simulink model "ACFT"  (R2024b)
settings: Solver=VariableStepAuto  StartTime=0.0  StopTime=10.0  RelTol=1e-3
values from neighbouring files (symbols this model uses):
  alfa_deg = -1.8    [initACFT_high.m]    (also in init_Cessna.m = 1)
  b = params.b    [Aerodynamics_Coefficient.m]    (also in AeroforcesandMoments.m; initACFT_high.m = 21; initACFT_low.m = 21; init_Cessna.m = 10.9728)
  c = params.c    [Aerodynamics_Coefficient.m]    (also in AeroforcesandMoments.m; initACFT_high.m = 2.5; initACFT_low.m = 2.5; init_Cessna.m = 1.49352)
  CD0 = params.CD0    [Aerodynamics_Coefficient.m]    (also in initACFT_high.m = 0.0281; initACFT_low.m = 0.023; init_Cessna.m = 0.027)
  CD_alpha = params.CD_alpha    [Aerodynamics_Coefficient.m]    (also in initACFT_high.m = 0.5157; initACFT_low.m = 0.1318; init_Cessna.m = 0.26)
  CD_elev = params.CD_elev    [Aerodynamics_Coefficient.m]    (also in initACFT_high.m = 0.0178; initACFT_low.m = 0.0178; init_Cessna.m = 0)
  CI_beta = params.CI_beta    [Aerodynamics_Coefficient.m]
  CI_p = params.CI_p    [Aerodynamics_Coefficient.m]
  CI_r = params.CI_r    [Aerodynamics_Coefficient.m]
  CI_rud = params.CI_rud    [Aerodynamics_Coefficient.m]
  CL0 = params.CL0    [Aerodynamics_Coefficient.m]    (also in initACFT_high.m = 0.209; initACFT_low.m = 0.19; init_Cessna.m = 0.307)
  CL_alpha = params.CL_alpha    [Aerodynamics_Coefficient.m]    (also in initACFT_high.m = 8.7491; initACFT_low.m = 6.1879; init_Cessna.m = 4.41)
  CL_elev = params.CL_elev    [Aerodynamics_Coefficient.m]    (also in initACFT_high.m = 0.538; initACFT_low.m = 0.4727; init_Cessna.m = 0.43)
  CL_q = params.CL_q    [Aerodynamics_Coefficient.m]    (also in initACFT_high.m = 4.14; initACFT_low.m = 4.66; init_Cessna.m = 3.9)
  Cm0 = params.Cm0    [Aerodynamics_Coefficient.m]    (also in initACFT_high.m = 0; initACFT_low.m = 0.0133; init_Cessna.m = 0.04)
  Cm_alpha = params.Cm_alpha    [Aerodynamics_Coefficient.m]    (also in initACFT_high.m = -2.4351; initACFT_low.m = -2.0168; init_Cessna.m = -0.613)
  Cm_AlphaDot = params.Cm_AlphaDot    [Aerodynamics_Coefficient.m]    (also in initACFT_high.m = -4.53; initACFT_low.m = -6.76; init_Cessna.m = -7.27)
  Cm_elev = params.Cm_elev    [Aerodynamics_Coefficient.m]    (also in initACFT_high.m = -1.9079; initACFT_low.m = -1.6788; init_Cessna.m = -1.122)
  Cm_q = params.Cm_q    [Aerodynamics_Coefficient.m]    (also in initACFT_high.m = -37.6; initACFT_low.m = -36.3; init_Cessna.m = -12.4)
  Cn_ail = -8.5944e-04    (= -0.00085944)    [initACFT_high.m]    (also in initACFT_low.m = -0.00063025; init_Cessna.m = -0.0216)
  Cn_beta = 0.1478    [initACFT_high.m]    (also in initACFT_low.m = 0.1209; init_Cessna.m = 0.0587)
  Cn_p = -0.114    [initACFT_high.m]    (also in initACFT_low.m; init_Cessna.m = -0.0278)
  Cn_r = -0.15    [initACFT_high.m]    (also in initACFT_low.m = -0.3; init_Cessna.m = -0.0937)
  Cn_rud = -0.1100    (= -0.11)    [initACFT_high.m]    (also in initACFT_low.m = -0.102; init_Cessna.m = -0.0645)
  CY_ail = 0    [initACFT_high.m]    (also in initACFT_low.m; init_Cessna.m)
  CY_beta = params.CY_beta    [Aerodynamics_Coefficient.m]    (also in initACFT_high.m = -1.2777; initACFT_low.m = -1.1803; init_Cessna.m = -0.404)
  CY_p = params.CY_p    [Aerodynamics_Coefficient.m]    (also in initACFT_high.m = 0.3; initACFT_low.m = 0.3; init_Cessna.m = -0.075)
  CY_r = params.CY_r    [Aerodynamics_Coefficient.m]    (also in initACFT_high.m = 0.91; initACFT_low.m = 0.91; init_Cessna.m = 0.214)
  CY_rud = params.CY_rud    [Aerodynamics_Coefficient.m]    (also in initACFT_high.m = 0.4343; initACFT_low.m = 0.4016; init_Cessna.m = 0.187)
  Inertia = [Ixx 0 -Ixz; 0 Iyy 0; -Ixz 0 Izz]    [initACFT_high.m]    (also in initACFT_low.m; init_Cessna.m)
  nrho = 0.75    [initACFT_high.m]    (also in initACFT_low.m; init_Cessna.m)
  nv = 0    [initACFT_high.m]    (also in initACFT_low.m; init_Cessna.m = -1)
  rho_reference_kgpm3 = 1.225    [initACFT_high.m]    (also in init_Cessna.m)
  S = 45    [initACFT_high.m]    (also in initACFT_low.m; init_Cessna.m = 16.2)
  V_reference_mps = 200    [initACFT_high.m]    (also in init_Cessna.m = 51.4)
  xf_m = -3.8    [initACFT_high.m]    (also in initACFT_low.m; init_Cessna.m = 1)
  z_cg = -0.4    [initACFT_high.m]    (also in initACFT_low.m; init_Cessna.m = 0.2)
  zf_m = -0.6    [initACFT_high.m]    (also in initACFT_low.m; init_Cessna.m = 0)
undefined symbols (not defined in the file or in its folder): CI_ail, CL_AlphaDot_, TMax, Y_cg, Z_cg

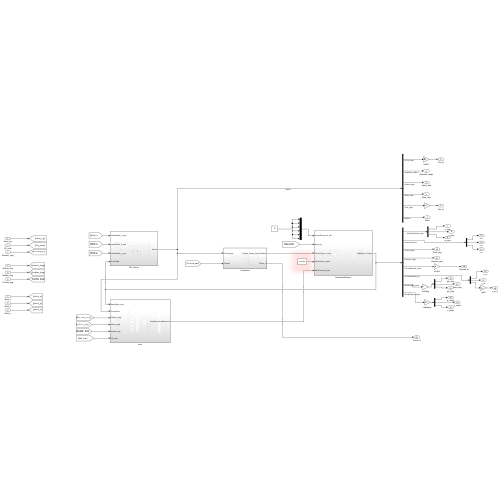
[thumbnail: Simulink's stored preview of the top-level diagram]
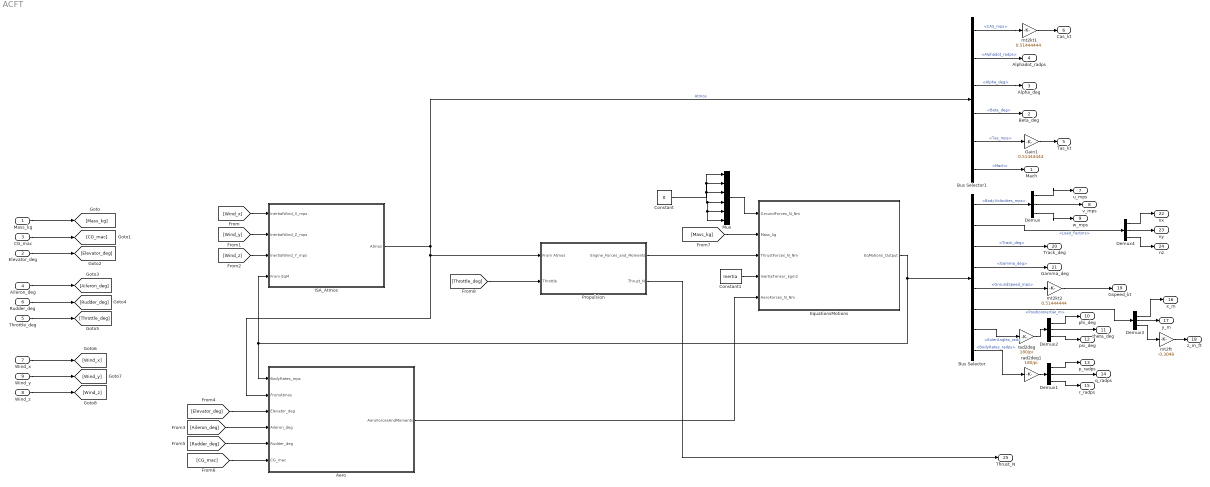
== system ACFT ==
  Mass_kg : Inport
  Elevator_deg : Inport  Port=2
  CG_mac : Inport  Port=3
  Aileron_deg : Inport  Port=4
  Throttle_deg : Inport  Port=5
  Rudder_deg : Inport  Port=6
  Wind_x : Inport  Port=7
  Wind_z : Inport  Port=8
  Wind_y : Inport  Port=9
  Aero : Subsystem
  Bus Selector : BusSelector  OutputSignals=BodyVolocities_mps,Load_Factors,Track_deg,Gamma_deg,GroundSpeed_mps,PositionInertial_m,EulerAngles_rad,BodyRates_radps
  Bus Selector1 : BusSelector  OutputSignals=CAS_mps,Alphadot_radps,Alpha_deg,Beta_deg,Tas_mps,Mach
  Constant : Constant  Value=0
  Constant1 : Constant  Value=Inertia
  Demux{,1..4} (5 alike) : Demux  Outputs=3
  EquationsMotions : Subsystem
  Gain1 : Gain  Gain=0.51444444
  ISA_Atmos : Subsystem
  Mux : Mux  Inputs=6
  Propulsion : Subsystem
  mt2ft : Gain  Gain=-0.3048
  mt2kt1 : Gain  Gain=0.51444444
  mt2kt2 : Gain  Gain=0.51444444
  rad2deg : Gain  Gain=180/pi
  rad2deg1 : Gain  Gain=180/pi
  Mach : Outport
  Beta_deg : Outport  Port=2
  Alpha_deg : Outport  Port=3
  Alphadot_radps : Outport  Port=4
  Tas_kt : Outport  Port=5
  Cas_kt : Outport  Port=6
  u_mps : Outport  Port=7
  v_mps : Outport  Port=8
  w_mps : Outport  Port=9
  phi_deg : Outport  Port=10
  theta_deg : Outport  Port=11
  psi_deg : Outport  Port=12
  p_radps : Outport  Port=13
  q_radps : Outport  Port=14
  r_radps : Outport  Port=15
  x_m : Outport  Port=16
  y_m : Outport  Port=17
  z_m_ft : Outport  Port=18
  Gspeed_kt : Outport  Port=19
  Track_deg : Outport  Port=20
  Gamma_deg : Outport  Port=21
  nx : Outport  Port=22
  ny : Outport  Port=23
  nz : Outport  Port=24
  Thrust_N : Outport  Port=25
  wires:
  EquationsMotions/1(EqMotions_Output) -> Aero/1(BodyRates_mps), ISA_Atmos/4(From EqM), Bus Selector/1
  ISA_Atmos/1(Atmos) -> Aero/2(FromAtmos), Propulsion/1(From Atmos), Bus Selector1/1  "Atmos"
  Aero/1(AeroForcesAndMoments) -> EquationsMotions/5(AeroForces_N_Nm)
  Propulsion/2(Thrust_N) -> Thrust_N/1
  Constant/1 -> Mux/1, Mux/6, Mux/5, Mux/4, Mux/3, Mux/2
  Mux/1 -> EquationsMotions/1(GroundForces_N_Nm)
  Constant1/1 -> EquationsMotions/4(InertiaTensor_kgm2)
  CG_mac/1 -> [CG_mac]
  Aileron_deg/1 -> [Aileron_deg]
  Rudder_deg/1 -> [Rudder_deg]
  Wind_x/1 -> [Wind_x]
  Wind_y/1 -> [Wind_y]
  Wind_z/1 -> [Wind_z]
  Throttle_deg/1 -> [Throttle_deg]
  Elevator_deg/1 -> [Elevator_deg]
  Mass_kg/1 -> [Mass_kg]
  [Wind_x] -> ISA_Atmos/1(InertialWind_X_mps)
  [Wind_y] -> ISA_Atmos/2(InertialWind_Z_mps)
  [Wind_z] -> ISA_Atmos/3(InertialWind_Y_mps)
  [Aileron_deg] -> Aero/4(Aileron_deg)
  [Elevator_deg] -> Aero/3(Elevator_deg)
  [Rudder_deg] -> Aero/5(Rudder_deg)
  [CG_mac] -> Aero/6(CG_mac)
  [Mass_kg] -> EquationsMotions/2(Mass_kg)
  [Throttle_deg] -> Propulsion/2(Throttle)
  Bus Selector1/1 -> mt2kt1/1  "<CAS_mps>"
  Bus Selector1/2 -> Alphadot_radps/1  "<Alphadot_radps>"
  Bus Selector1/3 -> Alpha_deg/1  "<Alpha_deg>"
  Bus Selector1/4 -> Beta_deg/1  "<Beta_deg>"
  Bus Selector1/5 -> Gain1/1  "<Tas_mps>"
  Bus Selector1/6 -> Mach/1  "<Mach>"
  Gain1/1 -> Tas_kt/1
  mt2kt1/1 -> Cas_kt/1
  Bus Selector/1 -> Demux/1  "<BodyVolocities_mps>"
  Bus Selector/3 -> Track_deg/1  "<Track_deg>"
  Bus Selector/4 -> Gamma_deg/1  "<Gamma_deg>"
  Bus Selector/6 -> Demux3/1  "<PositionInertial_m>"
  Bus Selector/7 -> rad2deg/1  "<EulerAngles_rad>"
  Bus Selector/8 -> rad2deg1/1  "<BodyRates_radps>"
  rad2deg/1 -> Demux2/1
  rad2deg1/1 -> Demux1/1
  Demux/1 -> u_mps/1
  Demux/3 -> w_mps/1
  Demux/2 -> v_mps/1
  Demux2/2 -> theta_deg/1
  Demux2/1 -> phi_deg/1
  Demux2/3 -> psi_deg/1
  Demux1/1 -> p_radps/1
  Demux1/3 -> r_radps/1
  Demux1/2 -> q_radps/1
  Demux3/2 -> y_m/1
  Demux3/1 -> x_m/1
  Demux3/3 -> mt2ft/1
  mt2ft/1 -> z_m_ft/1
  Bus Selector/5 -> mt2kt2/1  "<GroundSpeed_mps>"
  mt2kt2/1 -> Gspeed_kt/1
  Bus Selector/2 -> Demux4/1  "<Load_Factors>"
  Demux4/1 -> nx/1
  Demux4/3 -> nz/1
  Demux4/2 -> ny/1
  Propulsion/1(Engine_Forces_and_Moments) -> EquationsMotions/3(ThrustForces_N_Nm)

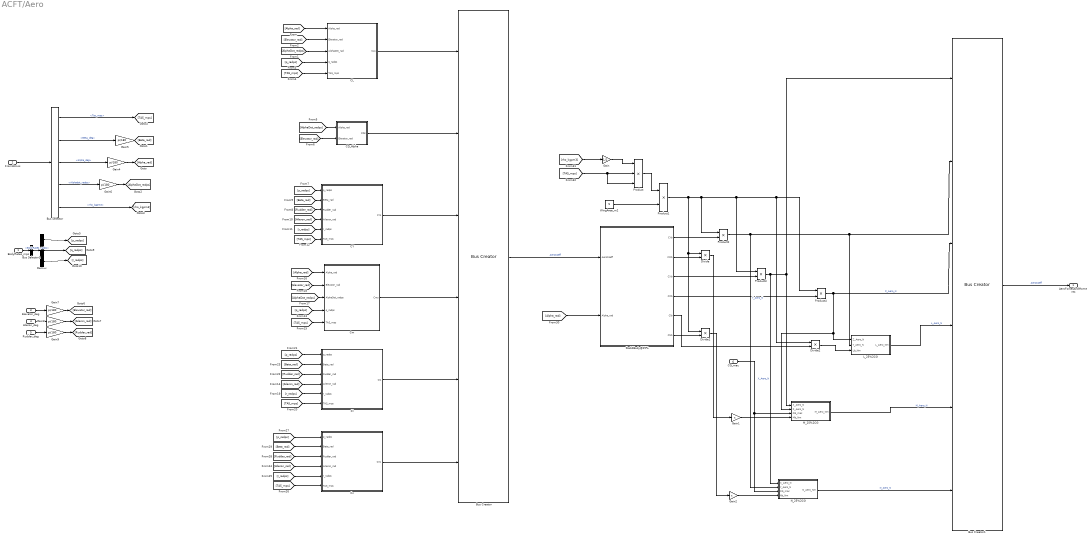
== system ACFT/Aero ==
  BodyRates_mps : Inport
  FromAtmos : Inport  Port=2
  Elevator_deg : Inport  Port=3
  Aileron_deg : Inport  Port=4
  Rudder_deg : Inport  Port=5
  CG_mac : Inport  Port=6
  Bus Creator : BusCreator  Inputs=6
  Bus Creator1 : BusCreator  Inputs=6
  Bus Selector : BusSelector  OutputSignals=Tas_mps,Beta_deg,Alpha_deg,Alphadot_radps,rho_kgpm3
  Bus Selector1 : BusSelector  OutputSignals=BodyRates_radps
  CD_Alpha : Subsystem
  CI : Subsystem
  CL : Subsystem
  CY : Subsystem
  Cm : Subsystem
  Cn : Subsystem
  Demux : Demux  Outputs=3
  Divide : Product
  Divide1 : Product
  Divide2 : Product
  Gain : Gain  Gain=1/2
  Gain1 : Gain  Gain=c
  Gain2 : Gain  Gain=c
  Gain{4..9} (6 alike) : Gain  Gain=pi/180
  L_25%2CG : Subsystem
  M_25%2CG : Subsystem
  N_25%2CG : Subsystem
  Product : Product  Inputs=3
  Product{1..4} (4 alike) : Product
  Stab2Body@25% : Subsystem
  WingArea_m2 : Constant  Value=S
  AeroForcesAndMoments : Outport
  wires:
  [p_radps] -> Cn/1(p_radps)
  [r_radps] -> CI/5(r_radps)
  Stab2Body@25%/2(CMb) -> Divide/2
  Stab2Body@25%/5(Clb) -> Divide2/2
  [rho_kgpm3] -> Gain/1
  Gain7/1 -> [Elevator_rad]
  Gain6/1 -> [AlphaDot_radps]
  CL/1(CLs) -> Bus Creator/1
  [TAS_mps] -> Cn/6(TAS_mps)
  [AlphaDot_radps] -> CL/3(AlphaDot_rad)
  N_25%2CG/1(N_Aero_Nm) -> Bus Creator1/6  "N_Aero_N"
  CI/1(CIs) -> Bus Creator/5
  M_25%2CG/1(M_Aero_Nm) -> Bus Creator1/5  "M_Aero_N"
  [p_radps] -> CY/1(p_radps)
  Stab2Body@25%/4(CZb) -> Product4/2
  [Alpha_rad] -> CL/1(Alpha_rad)
  [Aileron_rad] -> CI/4(Aileron_rad)
  Gain5/1 -> [Beta_rad]
  Cm/1(Cms) -> Bus Creator/4
  Gain2/1 -> N_25%2CG/4(Nb_Nm)
  [Beta_rad] -> CY/2(Beta_rad)
  Product2/1 -> L_25%2CG/2(Y_Aero_N), Bus Creator1/2, N_25%2CG/2(Y_Aero_N)  "Y_Aero_N"
  Elevator_deg/1 -> Gain7/1
  Gain/1 -> Product/1
  [Aileron_rad] -> Cn/4(Aileron_rad)
  CG_mac/1 -> M_25%2CG/3(CG_mac), N_25%2CG/3(CG_mac)
  [Rudder_rad] -> Cn/3(Rudder_rad)
  Demux/2 -> [q_radps]
  CD_Alpha/1(CDs) -> Bus Creator/2
  Demux/1 -> [p_radps]
  [TAS_mps] -> Cm/5(TAS_mps)
  [TAS_mps] -> Product/2, Product/3
  L_25%2CG/1(L_Aero_Nm) -> Bus Creator1/4  "L_Aero_N"
  Demux/3 -> [r_radps]
  CY/1(CYs) -> Bus Creator/3
  [AlphaDot_radps] -> Cm/3(AlphaDot_radps)
  [Rudder_rad] -> CI/3(Rudder_rad)
  [p_radps] -> CI/1(p_radps)
  [Rudder_rad] -> CY/3(Rudder_rad)
  Product1/1 -> Divide2/1, Product4/1, Product3/1, Product2/1, Divide/1, Divide1/1
  Gain1/1 -> M_25%2CG/4(Mb_Nm)
  Product4/1 -> Bus Creator1/3, L_25%2CG/1(Z_Aero_N), M_25%2CG/2(Z_Aero_N)  "Z_Aero_N"
  [Elevator_rad] -> Cm/2(Elevator_rad)
  Divide2/1 -> L_25%2CG/3(Lb_Nm)
  Gain9/1 -> [Rudder_rad]
  Aileron_deg/1 -> Gain8/1
  [Alpha_rad] -> Cm/1(Alpha_rad)
  Gain8/1 -> [Aileron_rad]
  [Beta_rad] -> Cn/2(Beta_rad)
  [Elevator_rad] -> CD_Alpha/2(Elevator_rad)
  Stab2Body@25%/1(CYb) -> Product2/2
  Rudder_deg/1 -> Gain9/1
  [Elevator_rad] -> CL/2(Elevator_rad)
  [Alpha_rad] -> Stab2Body@25%/2(Alpha_rad)
  Gain4/1 -> [Alpha_rad]
  Bus Creator/1 -> Stab2Body@25%/1(AeroCoeff)  "AeroCoeff"
  Stab2Body@25%/6(CNb) -> Divide1/2
  Cn/1(Cns) -> Bus Creator/6
  WingArea_m2/1 -> Product1/2
  [Aileron_rad] -> CY/4(Aileron_rad)
  [TAS_mps] -> CL/5(TAS_mps)
  Product/1 -> Product1/1
  Stab2Body@25%/3(CXb) -> Product3/2
  [AlphaDot_radps] -> CD_Alpha/1(Alpha_rad)
  Product3/1 -> Bus Creator1/1, M_25%2CG/1(X_Aero_N), N_25%2CG/1(X_Aero_N)  "X_Aero_N"
  [Beta_rad] -> CI/2(Beta_rad)
  [TAS_mps] -> CI/6(TAS_mps)
  [r_radps] -> CY/5(r_radps)
  Bus Creator1/1 -> AeroForcesAndMoments/1  "AeroCoeff"
  Divide1/1 -> Gain2/1
  [q_radps] -> Cm/4(q_radps)
  [TAS_mps] -> CY/6(TAS_mps)
  Divide/1 -> Gain1/1
  [r_radps] -> Cn/5(r_radps)
  [q_radps] -> CL/4(q_radps)
  FromAtmos/1 -> Bus Selector/1
  Bus Selector/2 -> Gain5/1  "<Beta_deg>"
  Bus Selector/3 -> Gain4/1  "<Alpha_deg>"
  Bus Selector/4 -> Gain6/1  "<Alphadot_radps>"
  Bus Selector/5 -> [rho_kgpm3]  "<rho_kgpm3>"
  Bus Selector/1 -> [TAS_mps]  "<Tas_mps>"
  BodyRates_mps/1 -> Bus Selector1/1
  Bus Selector1/1 -> Demux/1  "<BodyRates_radps>"

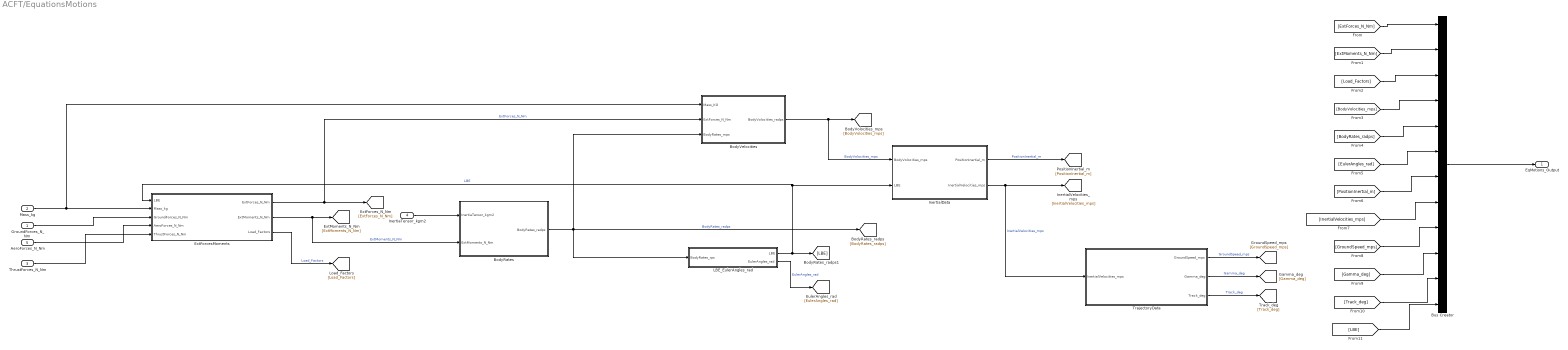
== system ACFT/EquationsMotions ==
  GroundForces_N_Nm : Inport
  Mass_kg : Inport  Port=2
  ThrustForces_N_Nm : Inport  Port=3
  InertiaTensor_kgm2 : Inport  Port=4
  AeroForces_N_Nm : Inport  Port=5
  BodyRates : Subsystem
  BodyVelocities : Subsystem
  Bus Creator : BusCreator  Inputs=12
  ExtForcesMoments : Subsystem
  InertialData : Subsystem
  LBE_EulerAngles_rad : Subsystem
  TrajectoryData : Subsystem
  EqMotions_Output : Outport
  wires:
  [Track_deg] -> Bus Creator/11
  [InertialVelocities_mps] -> Bus Creator/8
  [GroundSpeed_mps] -> Bus Creator/9
  [EulerAngles_rad] -> Bus Creator/6
  TrajectoryData/1(GroundSpeed_mps) -> [GroundSpeed_mps]  "GroundSpeed_mps"
  [Gamma_deg] -> Bus Creator/10
  TrajectoryData/2(Gamma_deg) -> [Gamma_deg]  "Gamma_deg"
  [ExtForces_N_Nm] -> Bus Creator/1
  TrajectoryData/3(Track_deg) -> [Track_deg]  "Track_deg"
  ExtForcesMoments/3(Load_Factors) -> [Load_Factors]  "Load_Factors"
  LBE_EulerAngles_rad/2(EulerAngles_rad) -> [EulerAngles_rad]  "EulerAngles_rad"
  InertialData/2(InertialVelocities_mps) -> [InertialVelocities_mps], TrajectoryData/1(InertialVelocities_mps)  "InertialVelocities_mps"
  [ExtMoments_N_Nm] -> Bus Creator/2
  BodyVelocities/1(BodyVolocities_radps) -> InertialData/1(BodyVolocities_mps), [BodyVolocities_mps]  "BodyVolocities_mps"
  ExtForcesMoments/2(ExtMoments_N_Nm) -> [ExtMoments_N_Nm], BodyRates/2(ExtMoments_N_Nm)  "ExtMoments_N_Nm"
  AeroForces_N_Nm/1 -> ExtForcesMoments/4(AeroForces_N_Nm)
  BodyRates/1(BodyRates_radps) -> BodyVelocities/3(BodyRates_mps), LBE_EulerAngles_rad/1(BodyRates_rps), [BodyRates_radps]  "BodyRates_radps"
  InertialData/1(PositionInertial_m) -> [PositionInertial_m]  "PositionInertial_m"
  Bus Creator/1 -> EqMotions_Output/1
  [BodyRates_radps] -> Bus Creator/5
  [PositionInertial_m] -> Bus Creator/7
  ThrustForces_N_Nm/1 -> ExtForcesMoments/5(ThrustForces_N_Nm)
  LBE_EulerAngles_rad/1(LBE) -> [LBE], InertialData/2(LBE), ExtForcesMoments/1(LBE)  "LBE"
  ExtForcesMoments/1(ExtForces_N_Nm) -> BodyVelocities/2(ExtForces_N_Nm), [ExtForces_N_Nm]  "ExtForces_N_Nm"
  [BodyVolocities_mps] -> Bus Creator/4
  InertiaTensor_kgm2/1 -> BodyRates/1(InertiaTensor_kgm2)
  GroundForces_N_Nm/1 -> ExtForcesMoments/3(GroundForces_N_Nm)
  Mass_kg/1 -> ExtForcesMoments/2(Mass_kg), BodyVelocities/1(Mass_KG)
  [Load_Factors] -> Bus Creator/3
  [LBE] -> Bus Creator/12

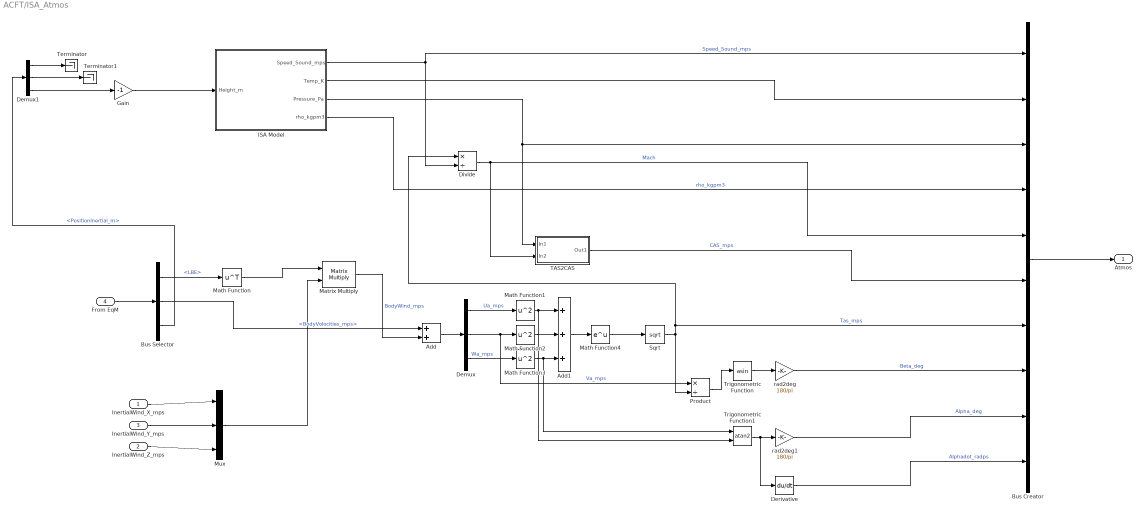
== system ACFT/ISA_Atmos ==
  InertialWind_X_mps : Inport
  InertialWind_Z_mps : Inport  Port=2
  InertialWind_Y_mps : Inport  Port=3
  From EqM : Inport  Port=4
  Add : Sum
  Add1 : Sum  Inputs=+++
  Bus Creator : BusCreator  Inputs=10
  Bus Selector : BusSelector  OutputSignals=LBE,BodyVolocities_mps,PositionInertial_m
  Demux : Demux  Outputs=3
  Demux1 : Demux  Outputs=3
  Derivative : Derivative
  Divide : Product  Inputs=*/
  Gain : Gain  Gain=-1
  ISA Model : Subsystem
  Math Function : Math  Operator=transpose
  Math Function1 : Math  Operator=square
  Math Function2 : Math  Operator=square
  Math Function3 : Math  Operator=square
  Math Function4 : Math
  Matrix Multiply : Product  Multiplication=Matrix(*)
  Mux : Mux  Inputs=3
  Product : Product  Inputs=*/
  Sqrt : Sqrt
  TAS2CAS : Subsystem
  Terminator : Terminator
  Terminator1 : Terminator
  Trigonometric Function : Trigonometry  Operator=asin
  Trigonometric Function1 : Trigonometry  Operator=atan2
  rad2deg : Gain  Gain=180/pi
  rad2deg1 : Gain  Gain=180/pi
  Atmos : Outport
  wires:
  Matrix Multiply/1 -> Add/2  "BodyWind_mps"
  Add/1 -> Demux/1
  Math Function4/1 -> Sqrt/1
  Divide/1 -> TAS2CAS/2(In2), Bus Creator/5  "Mach"
  Add1/1 -> Math Function4/1
  rad2deg/1 -> Bus Creator/8  "Beta_deg"
  Demux/1 -> Math Function1/1  "Ua_mps"
  ISA Model/4(rho_kgpm3) -> Bus Creator/4  "rho_kgpm3"
  From EqM/1 -> Bus Selector/1
  TAS2CAS/1(Out1) -> Bus Creator/6  "CAS_mps"
  Derivative/1 -> Bus Creator/10  "Alphadot_radps"
  Bus Creator/1 -> Atmos/1
  InertialWind_Z_mps/1 -> Mux/3
  Mux/1 -> Matrix Multiply/2
  Math Function/1 -> Matrix Multiply/1
  Trigonometric Function1/1 -> rad2deg1/1, Derivative/1
  ISA Model/3(Pressure_Pa) -> Bus Creator/3, TAS2CAS/1(In1)
  Math Function3/1 -> Add1/3, Trigonometric Function1/1
  ISA Model/1(Speed_Sound_mps) -> Bus Creator/1, Divide/2  "Speed_Sound_mps"
  InertialWind_Y_mps/1 -> Mux/2
  Sqrt/1 -> Product/2, Divide/1, Bus Creator/7  "Tas_mps"
  Math Function1/1 -> Add1/1, Trigonometric Function1/2
  ISA Model/2(Temp_K) -> Bus Creator/2
  Demux/3 -> Math Function3/1  "Wa_mps"
  Demux/2 -> Math Function2/1, Product/1  "Va_mps"
  Trigonometric Function/1 -> rad2deg/1
  InertialWind_X_mps/1 -> Mux/1
  Product/1 -> Trigonometric Function/1
  rad2deg1/1 -> Bus Creator/9  "Alpha_deg"
  Math Function2/1 -> Add1/2
  Bus Selector/1 -> Math Function/1  "<LBE>"
  Bus Selector/2 -> Add/1  "<BodyVolocities_mps>"
  Bus Selector/3 -> Demux1/1  "<PositionInertial_m>"
  Demux1/1 -> Terminator/1
  Demux1/2 -> Terminator1/1
  Demux1/3 -> Gain/1
  Gain/1 -> ISA Model/1(Height_m)

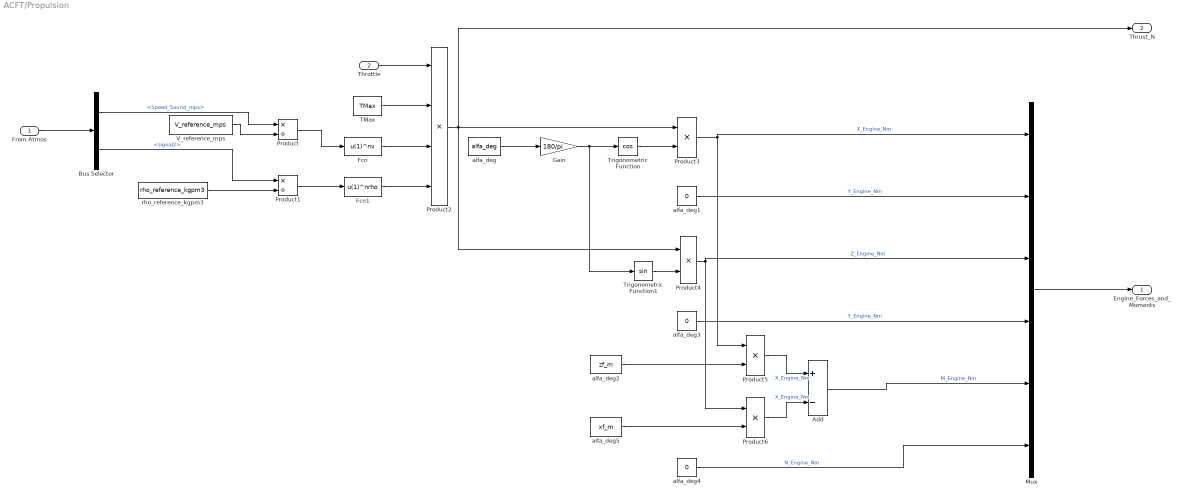
== system ACFT/Propulsion ==
  From Atmos : Inport
  Throttle : Inport  Port=2
  Add : Sum  Inputs=+-
  Bus Selector : BusSelector  OutputSignals=Speed_Sound_mps,signal2
  Fcn : Fcn  Expr=u(1)^nv
  Fcn1 : Fcn  Expr=u(1)^nrho
  Gain : Gain  Gain=180/pi
  Mux : Mux  Inputs=6
  Product : Product  Inputs=*/
  Product1 : Product  Inputs=*/
  Product2 : Product  Inputs=****
  Product{3..6} (4 alike) : Product
  TMax : Constant  Value=TMax
  Trigonometric Function : Trigonometry  Operator=cos
  Trigonometric Function1 : Trigonometry
  V_reference_mps : Constant  Value=V_reference_mps
  alfa_deg : Constant  Value=alfa_deg
  alfa_deg1 : Constant  Value=0
  alfa_deg2 : Constant  Value=zf_m
  alfa_deg3 : Constant  Value=0
  alfa_deg4 : Constant  Value=0
  alfa_deg5 : Constant  Value=xf_m
  rho_reference_kgpm3 : Constant  Value=rho_reference_kgpm3
  Engine_Forces_and_Moments : Outport
  Thrust_N : Outport  Port=2
  wires:
  alfa_deg/1 -> Gain/1
  alfa_deg1/1 -> Mux/2  "Y_Engine_Nm"
  Fcn/1 -> Product2/3
  Product3/1 -> Mux/1, Product5/1  "X_Engine_Nm"
  TMax/1 -> Product2/2
  alfa_deg3/1 -> Mux/4  "Y_Engine_Nm"
  Trigonometric Function1/1 -> Product4/2
  Fcn1/1 -> Product2/4
  Add/1 -> Mux/5  "M_Engine_Nm"
  alfa_deg4/1 -> Mux/6  "N_Engine_Nm"
  Bus Selector/2 -> Product1/1  "<signal2>"
  Gain/1 -> Trigonometric Function/1, Trigonometric Function1/1
  Bus Selector/1 -> Product/1  "<Speed_Sound_mps>"
  Product1/1 -> Fcn1/1
  From Atmos/1 -> Bus Selector/1
  Product4/1 -> Mux/3, Product6/1  "Z_Engine_Nm"
  Product/1 -> Fcn/1
  Product2/1 -> Product3/1, Product4/1, Thrust_N/1
  rho_reference_kgpm3/1 -> Product1/2
  Product6/1 -> Add/2  "X_Engine_Nm"
  Product5/1 -> Add/1  "X_Engine_Nm"
  Mux/1 -> Engine_Forces_and_Moments/1
  V_reference_mps/1 -> Product/2
  alfa_deg2/1 -> Product5/2
  alfa_deg5/1 -> Product6/2
  Trigonometric Function/1 -> Product3/2
  Throttle/1 -> Product2/1

== system ACFT/Aero/CD_Alpha ==
  Alpha_rad : Inport
  Elevator_rad : Inport  Port=2
  Abs : Abs  SaturateOnIntegerOverflow=off
  Abs1 : Abs  SaturateOnIntegerOverflow=off
  Add : Sum  Inputs=+++
  Constant : Constant  Value=CD0
  Gain : Gain  Gain=CD_alpha
  Gain1 : Gain  Gain=CD_elev
  CDs : Outport
  wires:
  Gain/1 -> Add/2
  Gain1/1 -> Add/3
  Elevator_rad/1 -> Abs1/1
  Add/1 -> CDs/1
  Abs/1 -> Gain/1
  Constant/1 -> Add/1
  Alpha_rad/1 -> Abs/1
  Abs1/1 -> Gain1/1

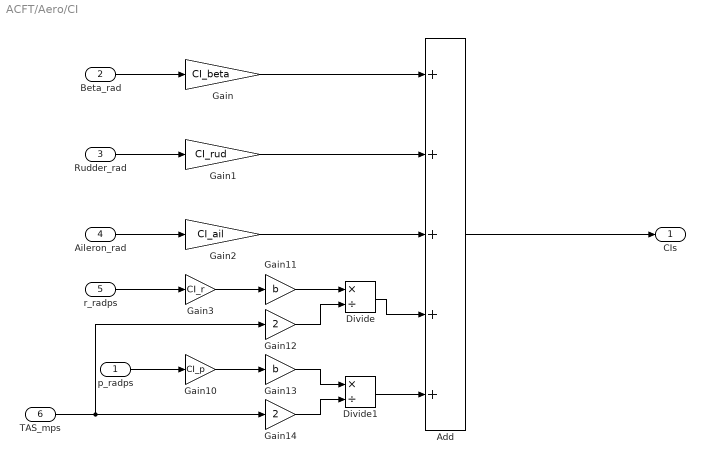
== system ACFT/Aero/CI ==
  p_radps : Inport
  Beta_rad : Inport  Port=2
  Rudder_rad : Inport  Port=3
  Aileron_rad : Inport  Port=4
  r_radps : Inport  Port=5
  TAS_mps : Inport  Port=6
  Add : Sum  Inputs=+++++
  Divide : Product  Inputs=*/
  Divide1 : Product  Inputs=*/
  Gain : Gain  Gain=CI_beta
  Gain1 : Gain  Gain=CI_rud
  Gain10 : Gain  Gain=CI_p
  Gain11 : Gain  Gain=b
  Gain12 : Gain  Gain=2
  Gain13 : Gain  Gain=b
  Gain14 : Gain  Gain=2
  Gain2 : Gain  Gain=CI_ail
  Gain3 : Gain  Gain=CI_r
  CIs : Outport
  wires:
  Divide1/1 -> Add/5
  r_radps/1 -> Gain3/1
  Beta_rad/1 -> Gain/1
  Aileron_rad/1 -> Gain2/1
  Gain1/1 -> Add/2
  p_radps/1 -> Gain10/1
  Divide/1 -> Add/4
  Gain10/1 -> Gain13/1
  TAS_mps/1 -> Gain14/1, Gain12/1
  Gain14/1 -> Divide1/2
  Gain11/1 -> Divide/1
  Gain12/1 -> Divide/2
  Add/1 -> CIs/1
  Gain2/1 -> Add/3
  Rudder_rad/1 -> Gain1/1
  Gain3/1 -> Gain11/1
  Gain/1 -> Add/1
  Gain13/1 -> Divide1/1

== system ACFT/Aero/CL ==
  Alpha_rad : Inport
  Elevator_rad : Inport  Port=2
  AlphaDot_rad : Inport  Port=3
  q_radps : Inport  Port=4
  TAS_mps : Inport  Port=5
  Add : Sum  Inputs=+++++
  Constant : Constant  Value=CL0
  Divide : Product  Inputs=*/
  Divide1 : Product  Inputs=*/
  Gain : Gain  Gain=CL_alpha
  Gain1 : Gain  Gain=CL_elev
  Gain2 : Gain  Gain=CL_AlphaDot_
  Gain3 : Gain  Gain=CL_q
  Gain4 : Gain  Gain=c
  Gain5 : Gain  Gain=2
  Gain6 : Gain  Gain=c
  Gain7 : Gain  Gain=2
  CLs : Outport
  wires:
  Gain7/1 -> Divide1/2
  Divide1/1 -> Add/4
  Gain6/1 -> Divide1/1
  Gain4/1 -> Divide/1
  Divide/1 -> Add/5
  Gain5/1 -> Divide/2
  TAS_mps/1 -> Gain5/1, Gain7/1
  Gain3/1 -> Gain4/1
  Add/1 -> CLs/1
  Gain2/1 -> Gain6/1
  Constant/1 -> Add/1
  Gain/1 -> Add/2
  Elevator_rad/1 -> Gain1/1
  Gain1/1 -> Add/3
  AlphaDot_rad/1 -> Gain2/1
  q_radps/1 -> Gain3/1
  Alpha_rad/1 -> Gain/1

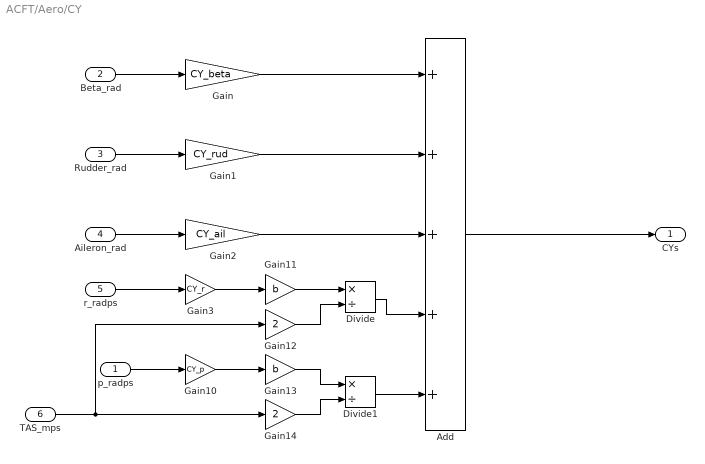
== system ACFT/Aero/CY ==
  p_radps : Inport
  Beta_rad : Inport  Port=2
  Rudder_rad : Inport  Port=3
  Aileron_rad : Inport  Port=4
  r_radps : Inport  Port=5
  TAS_mps : Inport  Port=6
  Add : Sum  Inputs=+++++
  Divide : Product  Inputs=*/
  Divide1 : Product  Inputs=*/
  Gain : Gain  Gain=CY_beta
  Gain1 : Gain  Gain=CY_rud
  Gain10 : Gain  Gain=CY_p
  Gain11 : Gain  Gain=b
  Gain12 : Gain  Gain=2
  Gain13 : Gain  Gain=b
  Gain14 : Gain  Gain=2
  Gain2 : Gain  Gain=CY_ail
  Gain3 : Gain  Gain=CY_r
  CYs : Outport
  wires:
  Divide1/1 -> Add/5
  r_radps/1 -> Gain3/1
  Beta_rad/1 -> Gain/1
  Aileron_rad/1 -> Gain2/1
  Gain1/1 -> Add/2
  p_radps/1 -> Gain10/1
  Divide/1 -> Add/4
  Gain10/1 -> Gain13/1
  TAS_mps/1 -> Gain14/1, Gain12/1
  Gain14/1 -> Divide1/2
  Gain11/1 -> Divide/1
  Gain12/1 -> Divide/2
  Add/1 -> CYs/1
  Gain2/1 -> Add/3
  Rudder_rad/1 -> Gain1/1
  Gain3/1 -> Gain11/1
  Gain/1 -> Add/1
  Gain13/1 -> Divide1/1

== system ACFT/Aero/Cm ==
  Alpha_rad : Inport
  Elevator_rad : Inport  Port=2
  AlphaDot_radps : Inport  Port=3
  q_radps : Inport  Port=4
  TAS_mps : Inport  Port=5
  Add : Sum  Inputs=+++++
  Constant : Constant  Value=Cm0
  Gain : Gain  Gain=Cm_alpha
  Gain1 : Gain  Gain=2
  Gain10 : Gain  Gain=Cm_AlphaDot
  Gain11 : Gain  Gain=c
  Gain12 : Gain  Gain=Cm_q
  Gain13 : Gain  Gain=2
  Gain2 : Gain  Gain=Cm_elev
  Gain3 : Gain  Gain=c
  Product : Product  Inputs=*/
  Product1 : Product  Inputs=*/
  Cms : Outport
  wires:
  Add/1 -> Cms/1
  Product/1 -> Add/4
  Gain/1 -> Add/2
  Gain11/1 -> Product1/1
  Gain10/1 -> Gain3/1
  q_radps/1 -> Gain12/1
  Gain12/1 -> Gain11/1
  Gain13/1 -> Product1/2
  Gain3/1 -> Product/1
  Product1/1 -> Add/5
  Alpha_rad/1 -> Gain/1
  Gain2/1 -> Add/3
  Gain1/1 -> Product/2
  TAS_mps/1 -> Gain13/1, Gain1/1
  Constant/1 -> Add/1
  Elevator_rad/1 -> Gain2/1
  AlphaDot_radps/1 -> Gain10/1

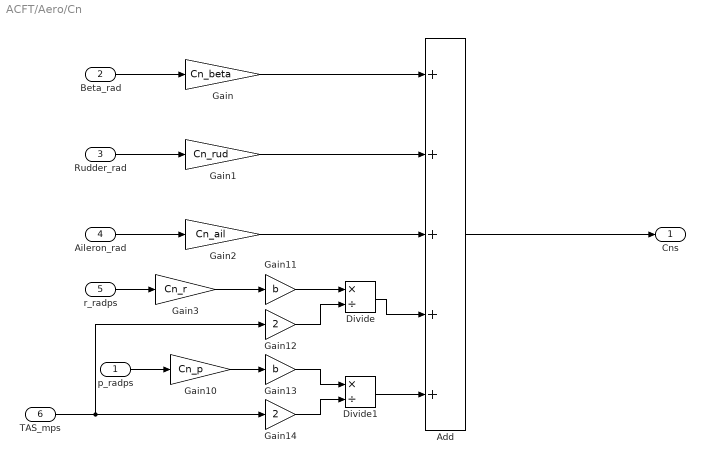
== system ACFT/Aero/Cn ==
  p_radps : Inport
  Beta_rad : Inport  Port=2
  Rudder_rad : Inport  Port=3
  Aileron_rad : Inport  Port=4
  r_radps : Inport  Port=5
  TAS_mps : Inport  Port=6
  Add : Sum  Inputs=+++++
  Divide : Product  Inputs=*/
  Divide1 : Product  Inputs=*/
  Gain : Gain  Gain=Cn_beta
  Gain1 : Gain  Gain=Cn_rud
  Gain10 : Gain  Gain=Cn_p
  Gain11 : Gain  Gain=b
  Gain12 : Gain  Gain=2
  Gain13 : Gain  Gain=b
  Gain14 : Gain  Gain=2
  Gain2 : Gain  Gain=Cn_ail
  Gain3 : Gain  Gain=Cn_r
  Cns : Outport
  wires:
  Divide1/1 -> Add/5
  r_radps/1 -> Gain3/1
  Beta_rad/1 -> Gain/1
  Aileron_rad/1 -> Gain2/1
  Gain1/1 -> Add/2
  p_radps/1 -> Gain10/1
  Divide/1 -> Add/4
  Gain10/1 -> Gain13/1
  TAS_mps/1 -> Gain14/1, Gain12/1
  Gain14/1 -> Divide1/2
  Gain11/1 -> Divide/1
  Gain12/1 -> Divide/2
  Add/1 -> Cns/1
  Gain2/1 -> Add/3
  Rudder_rad/1 -> Gain1/1
  Gain3/1 -> Gain11/1
  Gain/1 -> Add/1
  Gain13/1 -> Divide1/1

== system ACFT/Aero/L_25%2CG ==
  Z_Aero_N : Inport
  Y_Aero_N : Inport  Port=2
  Lb_Nm : Inport  Port=3
  Add : Sum  Inputs=+-+
  Constant : Constant  Value=z_cg
  Product5 : Product
  Product6 : Product
  Y_cg_m : Constant  Value=Y_cg
  L_Aero_Nm : Outport
  wires:
  Lb_Nm/1 -> Add/3
  Add/1 -> L_Aero_Nm/1  "L_Aero_Nm"
  Z_Aero_N/1 -> Product6/1
  Constant/1 -> Product5/2
  Y_Aero_N/1 -> Product5/1
  Y_cg_m/1 -> Product6/2
  Product5/1 -> Add/1
  Product6/1 -> Add/2

== system ACFT/Aero/M_25%2CG ==
  X_Aero_N : Inport
  Z_Aero_N : Inport  Port=2
  CG_mac : Inport  Port=3
  Mb_Nm : Inport  Port=4
  Add : Sum  Inputs=-++
  Fcn : Fcn  Expr=(u(1)-0.25)*c
  Product5 : Product
  Product6 : Product
  Z_cg_m : Constant  Value=Z_cg
  M_Aero_Nm : Outport
  wires:
  Mb_Nm/1 -> Add/3
  Add/1 -> M_Aero_Nm/1
  X_Aero_N/1 -> Product6/1
  Fcn/1 -> Product5/2
  Z_Aero_N/1 -> Product5/1
  Z_cg_m/1 -> Product6/2
  Product5/1 -> Add/1
  CG_mac/1 -> Fcn/1
  Product6/1 -> Add/2

== system ACFT/Aero/N_25%2CG ==
  X_Aero_N : Inport
  Y_Aero_N : Inport  Port=2
  CG_mac : Inport  Port=3
  Nb_Nm : Inport  Port=4
  Add : Sum  Inputs=+++
  Fcn : Fcn  Expr=(u(1)-0.25)*c
  Product5 : Product
  Product6 : Product
  Y_cg_m : Constant  Value=Y_cg
  N_Aero_Nm : Outport
  wires:
  Nb_Nm/1 -> Add/3
  Add/1 -> N_Aero_Nm/1  "N_Aero_Nm"
  X_Aero_N/1 -> Product6/1
  Fcn/1 -> Product5/2
  Y_Aero_N/1 -> Product5/1
  Y_cg_m/1 -> Product6/2
  Product5/1 -> Add/1
  CG_mac/1 -> Fcn/1
  Product6/1 -> Add/2

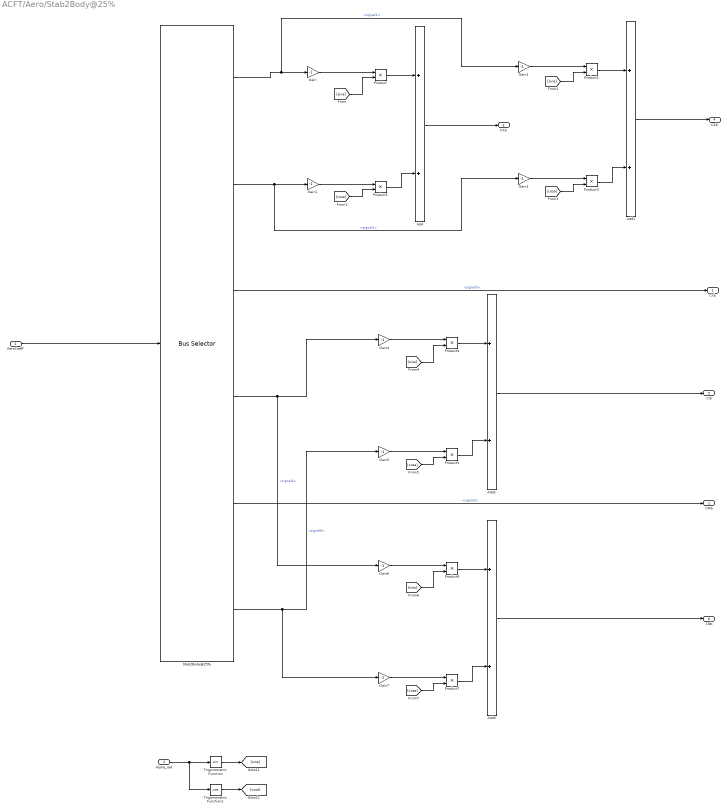
== system ACFT/Aero/Stab2Body@25% ==
  AeroCoeff : Inport
  Alpha_rad : Inport  Port=2
  Add{,1..3} (4 alike) : Sum
  Gain{,1..7} (8 alike) : Gain  Gain=-1
  Product{,1..7} (8 alike) : Product
  Stab2Body@25% : BusSelector  OutputSignals=signal1,signal2,signal3,signal4,signal5,signal6
  Trigonometric Function : Trigonometry
  Trigonometric Function1 : Trigonometry  Operator=cos
  CYb : Outport
  CMb : Outport  Port=2
  CXb : Outport  Port=3
  CZb : Outport  Port=4
  Clb : Outport  Port=5
  CNb : Outport  Port=6
  wires:
  Product7/1 -> Add3/2
  Product6/1 -> Add3/1
  Add3/1 -> CNb/1
  Gain7/1 -> Product7/1
  [cosa] -> Product7/2
  Gain6/1 -> Product6/1
  [sina] -> Product6/2
  [cosa] -> Product5/2
  Gain4/1 -> Product4/1
  Stab2Body@25%/4 -> Gain4/1, Gain6/1  "<signal4>"
  Product5/1 -> Add2/2
  Stab2Body@25%/6 -> Gain5/1, Gain7/1  "<signal6>"
  Add2/1 -> Clb/1
  [sina] -> Product4/2
  Gain5/1 -> Product5/1
  Product4/1 -> Add2/1
  [cosa] -> Product3/2
  Stab2Body@25%/2 -> Gain1/1, Gain3/1  "<signal2>"
  Gain2/1 -> Product2/1
  Product3/1 -> Add1/2
  Add1/1 -> CZb/1
  [sina] -> Product2/2
  Gain3/1 -> Product3/1
  Product2/1 -> Add1/1
  Add/1 -> CXb/1
  [cosa] -> Product1/2
  [sina] -> Product/2
  Gain1/1 -> Product1/1
  Gain/1 -> Product/1
  Product1/1 -> Add/2
  Product/1 -> Add/1
  Alpha_rad/1 -> Trigonometric Function/1, Trigonometric Function1/1
  Trigonometric Function1/1 -> [cosa]
  Trigonometric Function/1 -> [sina]
  Stab2Body@25%/1 -> Gain/1, Gain2/1  "<signal1>"
  Stab2Body@25%/3 -> CYb/1  "<signal3>"
  Stab2Body@25%/5 -> CMb/1  "<signal5>"
  AeroCoeff/1 -> Stab2Body@25%/1

== system ACFT/EquationsMotions/BodyRates ==
  InertiaTensor_kgm2 : Inport
  ExtMoments_N_Nm : Inport  Port=2
  CrossProduct : Subsystem
  Demux : Demux  Outputs=3
  Mux : Mux  Inputs=3
  Product : Product  Multiplication=Matrix(*)
  Product1 : Product  Inputs=/*
  Sum : Sum  Inputs=-+
  p_radps : Integrator
  q_radps : Integrator
  r_radps : Integrator
  BodyRates_radps : Outport
  wires:
  Mux/1 -> CrossProduct/1(A), Product/2, BodyRates_radps/1
  ExtMoments_N_Nm/1 -> Sum/2
  p_radps/1 -> Mux/1
  CrossProduct/1(C) -> Sum/1
  InertiaTensor_kgm2/1 -> Product/1, Product1/1
  Product/1 -> CrossProduct/2(B)
  Sum/1 -> Product1/2
  Demux/1 -> p_radps/1
  q_radps/1 -> Mux/2
  Demux/3 -> r_radps/1
  Product1/1 -> Demux/1
  Demux/2 -> q_radps/1
  r_radps/1 -> Mux/3

== system ACFT/EquationsMotions/BodyVelocities ==
  Mass_KG : Inport
  ExtForces_N_Nm : Inport  Port=2
  BodyRates_mps : Inport  Port=3
  Demux : Demux  Outputs=3
  Mux : Mux  Inputs=3
  Product : Product  Inputs=*/
  Sum : Sum  Inputs=|+-
  q_mps : Integrator
  u_mps : Integrator
  v_mps : Integrator
  BodyVolocities_radps : Outport
  wires:
  ExtForces_N_Nm/1 -> Product/1
  BodyRates_mps/1 -> Sum/2
  Sum/1 -> Demux/1
  v_mps/1 -> Mux/2
  Product/1 -> Sum/1
  Mass_KG/1 -> Product/2
  Demux/2 -> v_mps/1
  u_mps/1 -> Mux/1
  Demux/3 -> q_mps/1
  Demux/1 -> u_mps/1
  Mux/1 -> BodyVolocities_radps/1
  q_mps/1 -> Mux/3

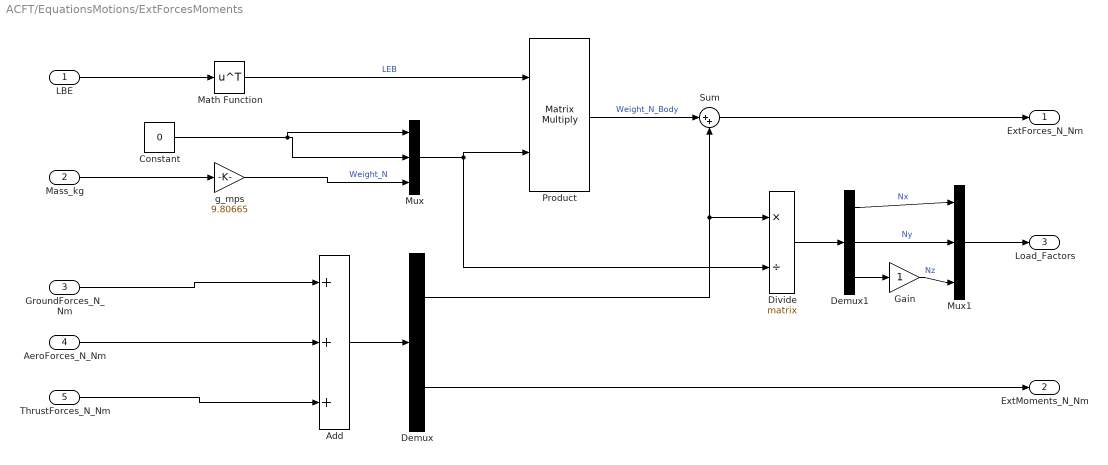
== system ACFT/EquationsMotions/ExtForcesMoments ==
  LBE : Inport
  Mass_kg : Inport  Port=2
  GroundForces_N_Nm : Inport  Port=3
  AeroForces_N_Nm : Inport  Port=4
  ThrustForces_N_Nm : Inport  Port=5
  Add : Sum  Inputs=+++
  Constant : Constant  Value=0
  Demux : Demux  Outputs=2
  Demux1 : Demux  Outputs=3
  Divide : Product  Inputs=*/  Multiplication=Matrix(*)
  Gain : Gain
  Math Function : Math  Operator=transpose
  Mux : Mux  Inputs=3
  Mux1 : Mux  Inputs=3
  Product : Product  Multiplication=Matrix(*)
  Sum : Sum  Inputs=|++
  g_mps : Gain  Gain=9.80665
  ExtForces_N_Nm : Outport
  ExtMoments_N_Nm : Outport  Port=2
  Load_Factors : Outport  Port=3
  wires:
  Demux1/2 -> Mux1/2  "Ny"
  Demux1/3 -> Gain/1
  AeroForces_N_Nm/1 -> Add/2
  g_mps/1 -> Mux/3  "Weight_N"
  Math Function/1 -> Product/1  "LEB"
  Mux/1 -> Divide/2, Product/2
  Gain/1 -> Mux1/3  "Nz"
  Mass_kg/1 -> g_mps/1
  ThrustForces_N_Nm/1 -> Add/3
  Sum/1 -> ExtForces_N_Nm/1
  LBE/1 -> Math Function/1
  Demux/1 -> Divide/1, Sum/2
  Constant/1 -> Mux/1, Mux/2
  Add/1 -> Demux/1
  Divide/1 -> Demux1/1
  GroundForces_N_Nm/1 -> Add/1
  Demux/2 -> ExtMoments_N_Nm/1
  Demux1/1 -> Mux1/1  "Nx"
  Mux1/1 -> Load_Factors/1
  Product/1 -> Sum/1  "Weight_N_Body"

== system ACFT/EquationsMotions/InertialData ==
  BodyVolocities_mps : Inport
  LBE : Inport  Port=2
  Demux : Demux  Outputs=3
  Matrix Multiply : Product  Multiplication=Matrix(*)
  Mux : Mux  Inputs=3
  XI_m : Integrator
  YI_m : Integrator
  ZI_m : Integrator
  PositionInertial_m : Outport
  InertialVelocities_mps : Outport  Port=2
  wires:
  Mux/1 -> PositionInertial_m/1
  LBE/1 -> Matrix Multiply/1
  BodyVolocities_mps/1 -> Matrix Multiply/2
  Demux/2 -> YI_m/1
  YI_m/1 -> Mux/2
  ZI_m/1 -> Mux/3
  Matrix Multiply/1 -> Demux/1, InertialVelocities_mps/1  "InertialVelocities_mps"
  Demux/1 -> XI_m/1
  Demux/3 -> ZI_m/1
  XI_m/1 -> Mux/1

== system ACFT/EquationsMotions/LBE_EulerAngles_rad ==
  BodyRates_rps : Inport
  Demux : Demux  Outputs=3
  EulerRates_radps : Subsystem
  LBE_rotation : Subsystem
  Mux : Mux  Inputs=3
  PHI_rad : Integrator
  PSI_rad : Integrator
  THETA_rad : Integrator
  LBE : Outport
  EulerAngles_rad : Outport  Port=2
  wires:
  Mux/1 -> LBE_rotation/1(EulerAngles_rad), EulerAngles_rad/1, EulerRates_radps/2(In2)
  EulerRates_radps/1(Out1) -> Demux/1
  BodyRates_rps/1 -> EulerRates_radps/1(BodyRates_rps)
  LBE_rotation/1(LBE) -> LBE/1
  Demux/3 -> PSI_rad/1
  Demux/1 -> PHI_rad/1
  THETA_rad/1 -> Mux/2
  PHI_rad/1 -> Mux/1
  PSI_rad/1 -> Mux/3
  Demux/2 -> THETA_rad/1

== system ACFT/EquationsMotions/TrajectoryData ==
  InertialVelocities_mps : Inport
  Add : Sum
  Demux : Demux  Outputs=3
  Gain : Gain  Gain=-1
  Gain1 : Gain  Gain=180*pi
  Gain2 : Gain  Gain=180*pi
  Math Function : Math  Operator=square
  Math Function1 : Math  Operator=square
  Sqrt : Sqrt
  Trigonometric Function : Trigonometry  Operator=atan2
  Trigonometric Function1 : Trigonometry  Operator=atan2
  GroundSpeed_mps : Outport
  Gamma_deg : Outport  Port=2
  Track_deg : Outport  Port=3
  wires:
  InertialVelocities_mps/1 -> Demux/1
  Trigonometric Function/1 -> Gain1/1
  Math Function1/1 -> Add/2
  Gain1/1 -> Gamma_deg/1
  Demux/2 -> Math Function1/1, Trigonometric Function1/2
  Demux/1 -> Math Function/1, Trigonometric Function1/1
  Gain2/1 -> Track_deg/1
  Gain/1 -> Trigonometric Function/1
  Math Function/1 -> Add/1
  Trigonometric Function1/1 -> Gain2/1
  Demux/3 -> Gain/1
  Sqrt/1 -> Trigonometric Function/2, GroundSpeed_mps/1
  Add/1 -> Sqrt/1

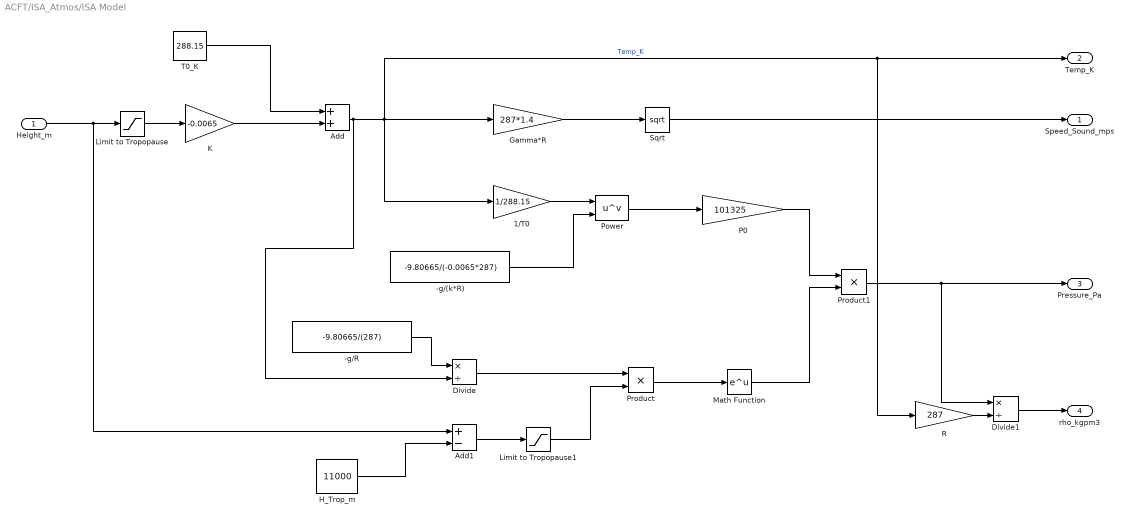
== system ACFT/ISA_Atmos/ISA Model ==
  Height_m : Inport
  -g/(k*R) : Constant  Value=-9.80665/(-0.0065*287)
  -g/R : Constant  Value=-9.80665/(287)
  1/T0 : Gain  Gain=1/288.15
  Add : Sum
  Add1 : Sum  Inputs=+-
  Divide : Product  Inputs=*/
  Divide1 : Product  Inputs=*/
  Gamma*R : Gain  Gain=287*1.4
  H_Trop_m : Constant  Value=11000
  K : Gain  Gain=-0.0065
  Limit to Tropopause : Saturate  UpperLimit=11000  LowerLimit=0
  Limit to Tropopause1 : Saturate  UpperLimit=inf  LowerLimit=0
  Math Function : Math
  P0 : Gain  Gain=101325
  Power : Math  Operator=pow
  Product : Product
  Product1 : Product
  R : Gain  Gain=287
  Sqrt : Sqrt
  T0_K : Constant  Value=288.15
  Speed_Sound_mps : Outport
  Temp_K : Outport  Port=2
  Pressure_Pa : Outport  Port=3
  rho_kgpm3 : Outport  Port=4
  wires:
  Product/1 -> Math Function/1
  Math Function/1 -> Product1/2
  Divide/1 -> Product/1
  P0/1 -> Product1/1
  K/1 -> Add/2
  Add/1 -> Divide/2, Gamma*R/1, 1/T0/1, Temp_K/1, R/1  "Temp_K"
  R/1 -> Divide1/2
  Divide1/1 -> rho_kgpm3/1
  Limit to Tropopause1/1 -> Product/2
  Product1/1 -> Divide1/1, Pressure_Pa/1
  Gamma*R/1 -> Sqrt/1
  H_Trop_m/1 -> Add1/2
  Add1/1 -> Limit to Tropopause1/1
  Sqrt/1 -> Speed_Sound_mps/1
  Height_m/1 -> Limit to Tropopause/1, Add1/1
  Power/1 -> P0/1
  -g/R/1 -> Divide/1
  Limit to Tropopause/1 -> K/1
  -g/(k*R)/1 -> Power/2
  1/T0/1 -> Power/1
  T0_K/1 -> Add/1

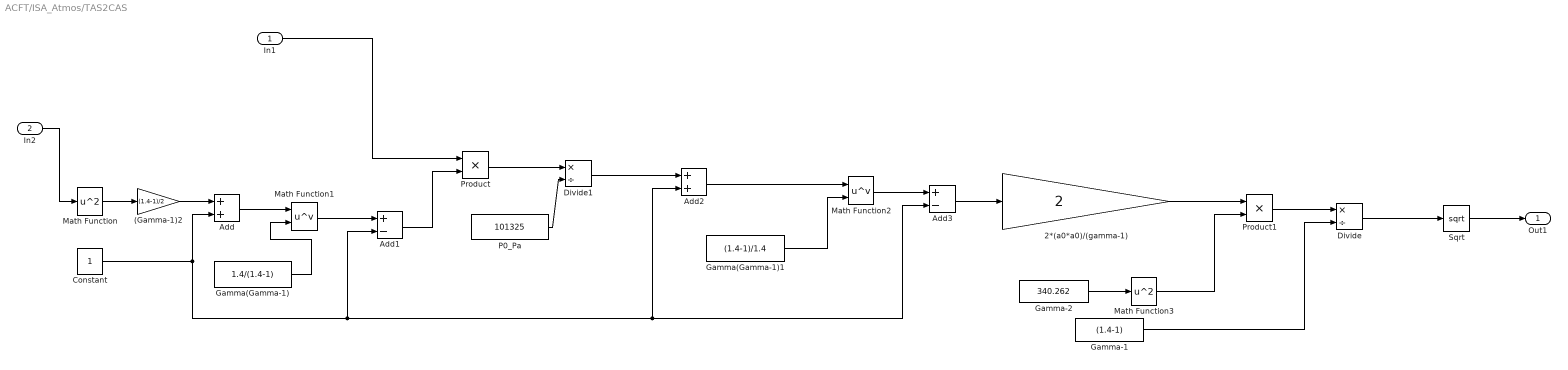
== system ACFT/ISA_Atmos/TAS2CAS ==
  In1 : Inport
  In2 : Inport  Port=2
  (Gamma-1)2 : Gain  Gain=(1.4-1)/2
  2*(a0*a0)/(gamma-1) : Gain  Gain=2
  Add : Sum
  Add1 : Sum  Inputs=+-
  Add2 : Sum
  Add3 : Sum  Inputs=+-
  Constant : Constant
  Divide : Product  Inputs=*/
  Divide1 : Product  Inputs=*/
  Gamma(Gamma-1) : Constant  Value=1.4/(1.4-1)
  Gamma(Gamma-1)1 : Constant  Value=(1.4-1)/1.4
  Gamma-1 : Constant  Value=(1.4-1)
  Gamma-2 : Constant  Value=340.262
  Math Function : Math  Operator=square
  Math Function1 : Math  Operator=pow
  Math Function2 : Math  Operator=pow
  Math Function3 : Math  Operator=square
  P0_Pa : Constant  Value=101325
  Product : Product
  Product1 : Product
  Sqrt : Sqrt
  Out1 : Outport
  wires:
  Product1/1 -> Divide/1
  Math Function3/1 -> Product1/2
  Gamma-2/1 -> Math Function3/1
  Divide/1 -> Sqrt/1
  Gamma-1/1 -> Divide/2
  In2/1 -> Math Function/1
  Product/1 -> Divide1/1
  Sqrt/1 -> Out1/1
  Math Function1/1 -> Add1/1
  Add3/1 -> 2*(a0*a0)/(gamma-1)/1
  Math Function2/1 -> Add3/1
  Gamma(Gamma-1)1/1 -> Math Function2/2
  Divide1/1 -> Add2/1
  Constant/1 -> Add/2, Add3/2, Add2/2, Add1/2
  Add2/1 -> Math Function2/1
  P0_Pa/1 -> Divide1/2
  2*(a0*a0)/(gamma-1)/1 -> Product1/1
  Gamma(Gamma-1)/1 -> Math Function1/2
  In1/1 -> Product/1
  Add/1 -> Math Function1/1
  Add1/1 -> Product/2
  (Gamma-1)2/1 -> Add/1
  Math Function/1 -> (Gamma-1)2/1

== system ACFT/EquationsMotions/BodyRates/CrossProduct ==
  A : Inport
  B : Inport  Port=2
  Add : Sum  Inputs=+-
  Demux : Demux  Outputs=3
  Demux1 : Demux  Outputs=3
  Mux : Mux  Inputs=3
  Mux1 : Mux  Inputs=3
  Product{,1..5} (6 alike) : Product
  C : Outport
  wires:
  Demux1/2 -> Product2/2, Product3/2
  Mux1/1 -> Add/2
  Add/1 -> C/1  "AxB"
  Demux1/1 -> Product1/2, Product5/2
  Demux1/3 -> Product/2, Product4/2
  Product3/1 -> Mux1/1
  Product2/1 -> Mux/3
  Product1/1 -> Mux/2
  Demux/3 -> Product1/1, Product3/1
  Demux/1 -> Product2/1, Product4/1
  Mux/1 -> Add/1
  Product4/1 -> Mux1/2
  Demux/2 -> Product/1, Product5/1
  Product/1 -> Mux/1
  A/1 -> Demux/1
  B/1 -> Demux1/1
  Product5/1 -> Mux1/3

== system ACFT/EquationsMotions/LBE_EulerAngles_rad/EulerRates_radps ==
  BodyRates_rps : Inport
  In2 : Inport  Port=2
  Abs : Abs  SaturateOnIntegerOverflow=off
  Constant : Constant  Value=0.001
  Demux : Demux  Outputs=3
  Divide : Product  Inputs=**
  Mux : Mux  Inputs=3
  Mux1 : Mux  Inputs=3
  Mux2 : Mux  Inputs=3
  Relay : Relay  OnSwitchValue=0.001  OffSwitchValue=0  OnOutputValue=0  OffOutputValue=1
  Sign : Signum
  Switch : Switch  Criteria=u2 > Threshold  SaturateOnIntegerOverflow=off  InputSameDT=off
  Trigonometric Function : Trigonometry  Operator=sincos
  phidot_radps2 : Fcn  Expr=u(1)+u(2)*u(4)*(u(5)/u(8))+u(3)*u(7)*(u(5)/u(8))
  psidot_radps2 : Fcn  Expr=(u(2)*u(5)+u(3)*u(7))/u(8)
  thetadot_radps2 : Fcn  Expr=u(2)*u(7)-u(3)*u(4)
  Out1 : Outport
  wires:
  psidot_radps2/1 -> Mux1/3
  Abs/1 -> Relay/1
  Trigonometric Function/2 -> Demux/1
  Relay/1 -> Switch/2
  Mux2/1 -> Mux/3
  thetadot_radps2/1 -> Mux1/2
  Mux/1 -> psidot_radps2/1, thetadot_radps2/1, phidot_radps2/1
  phidot_radps2/1 -> Mux1/1
  Demux/2 -> Sign/1, Abs/1, Switch/3
  Switch/1 -> Mux2/2
  Sign/1 -> Divide/2
  Constant/1 -> Divide/1
  Mux1/1 -> Out1/1
  In2/1 -> Trigonometric Function/1
  Trigonometric Function/1 -> Mux/2
  Demux/1 -> Mux2/1
  BodyRates_rps/1 -> Mux/1
  Demux/3 -> Mux2/3
  Divide/1 -> Switch/1

== system ACFT/EquationsMotions/LBE_EulerAngles_rad/LBE_rotation ==
  EulerAngles_rad : Inport
  Fcn : Fcn  Expr=u(5)*u(6)
  Fcn1 : Fcn  Expr=u(1)*u(2)*u(6)-u(4)*u(3)
  Fcn2 : Fcn  Expr=u(6)*u(2)*u(4)+u(1)*u(3)
  Fcn3 : Fcn  Expr=u(5)*u(3)
  Fcn4 : Fcn  Expr=u(1)*u(2)*u(3)+u(4)*u(6)
  Fcn5 : Fcn  Expr=u(4)*u(2)*u(3)-u(1)*u(6)
  Fcn6 : Fcn  Expr=u(4)*u(5)
  Fcn7 : Fcn  Expr=u(1)*u(5)
  Fcn8 : Fcn  Expr=-u(2)
  Math Function : Math  Operator=transpose
  Mux1 : Mux  Inputs=2
  Mux2 : Mux  Inputs=9
  Reshape : Reshape  OutputDimensionality=Customize  OutputDimensions=[3,1]
  Trigonometric Function : Trigonometry  Operator=sincos
  LBE : Outport
  wires:
  Mux2/1 -> Reshape/1
  Trigonometric Function/1 -> Mux1/1
  Fcn1/1 -> Mux2/2
  Fcn8/1 -> Mux2/7
  Fcn5/1 -> Mux2/6
  Reshape/1 -> Math Function/1
  EulerAngles_rad/1 -> Trigonometric Function/1
  Fcn7/1 -> Mux2/8
  Fcn/1 -> Mux2/1
  Math Function/1 -> LBE/1
  Fcn4/1 -> Mux2/5
  Mux1/1 -> Fcn/1, Fcn1/1, Fcn2/1, Fcn3/1, Fcn4/1, Fcn5/1, Fcn8/1, Fcn7/1, Fcn6/1
  Trigonometric Function/2 -> Mux1/2
  Fcn3/1 -> Mux2/4
  Fcn2/1 -> Mux2/3
  Fcn6/1 -> Mux2/9
